simulink model "SO3_model_AIS"  (R2022a)
settings: Solver=ode4  StartTime=0.0  StopTime=180  FixedStep=0.02  RelTol=1e-3
values from neighbouring files (symbols this model uses):
  alpha = 0.05    [Ini_SO3.m]    (also in Ini_SO3_MixedCZ.m = 0.3; coneNew.m = acos(cosalpha))
  alpha1 = 0.25    [Ini_SO3.m]
  beta = 0.05    [Ini_SO3.m]    (also in Ini_SO3_MixedCZ.m = 0.3)
  deltar = 0.005    [Ini_SO3.m]    (also in Ini_SO3_MixedCZ.m = 0.01; Ini_Usat.m = 0.01)
  G = [1,0,0 ... (first row only)    [Ini_SO3.m]    (also in Ini_SO3_MixedCZ.m; Symmetric test.m = inv(J)*D*E*D')
  J0 = [60 0 -5 ... (first row only)    [Ini_SO3.m]    (also in Ini_SO3_MixedCZ.m)
  J1 = [60 0 -5 ... (first row only)    [Ini_SO3.m]    (also in Ini_SO3_MixedCZ.m)
  J2 = [60 0 -5 ... (first row only)    [Ini_SO3.m]    (also in Ini_SO3_MixedCZ.m)
  J3 = [60 0 -5 ... (first row only)    [Ini_SO3.m]    (also in Ini_SO3_MixedCZ.m)
  K1 = [0.01,0,30,0.2]'    [Ini_SO3.m]    (also in Ini_SO3_MixedCZ.m = [0.01,0,30,0.1]')
  K2 = [0.01,55,55,16,0.001,0.001,0.001]'    [Ini_SO3.m]
  lambda = 0.05    [Ini_SO3.m]    (also in Ini_SO3_MixedCZ.m = 0.3; SO3toThetan.m = diag(lambda))
  lambda1 = 0.25    [Ini_SO3.m]
  N = R/deltar    (= 200)    [Ini_SO3.m]    (also in Ini_SO3_MixedCZ.m; Ini_Usat.m)
  Omega01 = [0.03;0.02;-0.03]    [Ini_SO3.m]    (also in Ini_SO3_MixedCZ.m = [0,0,0])
  Omega02 = [-0.02;0.02;-0.03]    [Ini_SO3.m]    (also in Ini_SO3_MixedCZ.m = [0,0,0])
  Omega03 = [0;0.03;0.04]    [Ini_SO3.m]    (also in Ini_SO3_MixedCZ.m = [0,0,0])
  Omega0d = [0;0;0]    [Ini_SO3.m]    (also in Ini_SO3_MixedCZ.m)
  R = 1    [Ini_SO3.m]    (also in Ini_SO3_MixedCZ.m = 2; Ini_Usat.m = 2; SO3.m = eye(3)+(1-cos(ang))*x2x_hat(x)*x2x_hat(x)+sin(ang)*x2x_hat(x; plot2D.m = tran(lamda_con(j),phi_con(j)))
  R01 = SO3(deg2rad(-80), nd0)    [Ini_SO3.m]    (also in Ini_SO3_MixedCZ.m = SO3(2.387, [0.3145,0.9113,0.2658]'))
  R02 = SO3(deg2rad(40),[0;1;1]/norm([0;1;1]))    [Ini_SO3.m]    (also in Ini_SO3_MixedCZ.m = SO3(1.422, [0.1772,0.9751,-0.1329]'))
  R03 = SO3(deg2rad(-120), nd0)    [Ini_SO3.m]    (also in Ini_SO3_MixedCZ.m = SO3(2.007, [0.2997,0.9415,0.1543]'))
  Rd = SO3(-(2*pi-Angd),nd)    [Ini_SO3.m]    (also in Ini_SO3_MixedCZ.m = SO3(Angd,nd))
  Rd0 = SO3(-(2*pi-Angd0),nd0)    [Ini_SO3.m]    (also in Ini_SO3_MixedCZ.m = SO3(Angd0,nd0))
  thate_T = deg2rad(30)    [Ini_SO3.m]    (also in Ini_SO3_MixedCZ.m = deg2rad(10))
  X = zeros(4,4)    [Ini_SO3.m]    (also in Ini_SO3_MixedCZ.m; coneNew.m = R .* cos(A))
undefined symbols (not defined in the file or in its folder): deg, rad, s
libraries: matrix_library x7, aerolibconvert2 x5
(part 2 of 2)

== matlab function SO3_model_AIS/Virtual leader/Controller1 ==
  settings: updateMethod=DISCRETE
  data: Rd input; Omegad input; Omega1 input; R1 input; R10 input; G input; ud output; X input; alpha input; lambda input; K input; J1 input; Psit1 output; theta output; t input; dot_Phi1 output; a data_store_memory; b data_store_memory; tel_Id output; ant_Id output
function [ud,Psit1,theta,dot_Phi1,tel_Id,ant_Id]  = fcn(Rd,Omegad,Omega1,R1,R10,G,X,alpha,lambda,K,J1,t)
% X = n*4, 4= 1*3+1;
ud=zeros(3,1);
global a;
global b;

    %% Attitude Error Function
    
    Psit1 =0.5*trace(G*(eye(3)-Rd'*R1));
    
    e_R1t = x_hat2x(G*Rd'*R1-R1'*Rd*G);
    
    e_omega_1=Omega1-R1'*Rd*Omegad;
    
%     if t>70
%        aa=R1;
%     end
%     
    %% Attitude Error Dynamics

%     dot_Psit1 = e_omega_1'*e_R1t;
    dot_Psit1 = e_R1t;
    
    %% Mixed attitude constraints
%     tel = [0.750,0.433,0.500]'; %telescope
    tel = [0,0,1]'; %telescope
    ant = [0,1,0]'; %antenna
%     aa= R1*ant;
    tel_Id = zeros(3,1);
    ant_Id = zeros(3,1);
    
    tel_Id = R1*tel;
    ant_Id = R1*ant;
    
    
    Phi1 = 1;
    dot_Phi1 = zeros(3,1);
    n=(size(X,1));
    theta=zeros(4,1);
%         Ang=deg2rad(10);
        flag=zeros(4,1);

        for i = 1:n
            if i<n % static attitude-forbidden zones
                theta(i)=rad2deg(acos(tel'*R1'*X(i,1:3)'));
                    if b(i)==0
                        if cos(X(i,end))-tel'*R10'*X(i,1:3)'>0
                            a(i)=0;
                        end
                        if cos(X(i,end))-tel'*R10'*X(i,1:3)'<=0
                            a(i)=1;
                            if cos(X(i,end))-tel'*R1'*X(i,1:3)'>0 && abs(alpha*(tel'*R1'*X(i,1:3)'-cos(pi))^2/2+alpha * log((cos(X(i,end))-tel'*R1'*X(i,1:3)')/(1+cos(X(i,end)))))<0.01
                            a(i)=0;
                            b(i)=1;
                            end
                        end
                    end
                    if a(i)==1
                        Phi1=Phi1+alpha*(tel'*R1'*X(i,1:3)'-cos(pi))^2/2;
                        dot_Phi1 = dot_Phi1+alpha*(tel'*R1'*X(i,1:3)'-cos(pi))*(x2x_hat(R1'*X(i,1:3)')*tel);
                    else
                        Phi1 = Phi1  + (-alpha * log((cos(X(i,end))-tel'*R1'*X(i,1:3)')/(1+cos(X(i,end)))));
                        dot_Phi1 = dot_Phi1 ...
                        + (alpha*(x2x_hat(R1'*X(i,1:3)')*tel)/(tel'*R1'*X(i,1:3)'-cos(X(i,end))));
                    end    
             end
   
             if i==n % the attitude-mandatory zones
                 theta(i)=rad2deg(acos(ant'*R1'*X(i,1:3)'));
                    if b(i)==0
                        if cos(X(i,end))-ant'*R10'*X(i,1:3)'<0
                            a(i)=0;
                        end
                        if cos(X(i,end))-ant'*R10'*X(i,1:3)'>=0
                            a(i)=1;
                            if cos(X(i,end))-ant'*R1'*X(i,1:3)'<0 && abs(lambda*(cos(0)-ant'*R1'*X(i,1:3)')^2/2-(-lambda * log((ant'*R1'*X(i,1:3)'-cos(X(i,end)))/(1+cos(X(i,end))))))<0.01
                            a(i)=0;
                            b(i)=1;
                            end
                        end
                    end
                    if a(i)==1
                        Phi1 = Phi1 + lambda*(cos(0)-ant'*R1'*X(i,1:3)')^2/2;
                        dot_Phi1 = dot_Phi1-lambda *(cos(0)-ant'*R1'*X(i,1:3)')*(x2x_hat(R1'*X(i,1:3)')*ant);
                    else
                        Phi1 = Phi1  + (-lambda * log((ant'*R1'*X(i,1:3)'-cos(X(i,end)))/(1+cos(X(i,end)))));
                        dot_Phi1 = dot_Phi1 ...
                            + (lambda*(x2x_hat(R1'*X(i,1:3)')*ant)/(ant'*R1'*X(i,1:3)'-cos(X(i,end))));
                    end
            end
        end

% if flag==0 
%% 传统不考虑饱和控制器 
%         for i = 1:n
%                 if i<n % static attitude-forbidden zones
%                          Phi1 = Phi1  + (-alpha * log((cos(X(i,end))-tel'*R1'*X(i,1:3)')/(1+cos(X(i,end)))));
%                         dot_Phi1 = dot_Phi1 ...
%                         + (alpha*(x2x_hat(R1'*X(i,1:3)')*tel)/(tel'*R1'*X(i,1:3)'-cos(X(i,end))));
%                     theta(i)=rad2deg(acos(tel'*R1'*X(i,1:3)'));
%                 end
%                  if i==n % the attitude-mandatory zones
%                     theta(i)=rad2deg(acos(ant'*R1'*X(i,1:3)'));
%                         Phi1 = Phi1  + (-lambda * log((ant'*R1'*X(i,1:3)'-cos(X(i,end)))/(1+cos(X(i,end)))));
%                         dot_Phi1 = dot_Phi1 ...
%                             + (lambda*(x2x_hat(R1'*X(i,1:3)')*ant)/(ant'*R1'*X(i,1:3)'-cos(X(i,end))));
%                  end
%         end
%      if t>=300
        ksi=0.001; % 滑模平滑项
        S1=Omega1/((norm(Omega1)^2)+ksi);
        ud=-K(1)*Psit1*S1-K(3)*Omega1-K(4)*(Psit1*dot_Phi1+e_R1t*Phi1);
%      else
%         ud=[0,0,0]';
%      end
end

== matlab function SO3_model_AIS/Input saturation3/Sliding Mode Control2 ==
  data: s input; dot_hat_beta output; u input; hat_beta input
function dot_hat_beta  = fcn(s,u,hat_beta)
    dot_hat_beta=zeros(3,1);
   
   k_beta=0.05;
   ksi3 =1.1;
   delta3=0.001;
   
   if hat_beta(1)^2<ksi3 || (hat_beta(1)^2>=ksi3 && -s(1)*u(1)*hat_beta(1)<0)
        dot_hat_beta(1) = -k_beta*s(1)*u(1);
   end
   if hat_beta(1)^2>=ksi3 && -s(1)*u(1)*hat_beta(1)>=0
        dot_hat_beta(1) = k_beta*(-s(1)*u(1)-(norm(hat_beta(1))^2-ksi3)*(-s(1)*u(1))*hat_beta(1)/(delta3*norm(hat_beta(1))^2)*hat_beta(1));
   end
   
   if hat_beta(2)^2<ksi3 || (hat_beta(2)^2>=ksi3 && -s(2)*u(2)*hat_beta(2)<0)
        dot_hat_beta(2) = -k_beta*s(2)*u(2);
   end
   if hat_beta(2)^2>=ksi3 && -s(2)*u(2)*hat_beta(2)>=0
        dot_hat_beta(2) = k_beta*(-s(2)*u(2)-(norm(hat_beta(2))^2-ksi3)*(-s(2)*u(2))*hat_beta(2)/(delta3*norm(hat_beta(2))^2)*hat_beta(2));
   end
   
   if hat_beta(3)^2<ksi3 || (hat_beta(3)^2>=ksi3 && -s(3)*u(3)*hat_beta(3)<0)
        dot_hat_beta(3) = -k_beta*s(3)*u(3);
   end
   if hat_beta(3)^2>=ksi3 && -s(3)*u(3)*hat_beta(3)>=0
        dot_hat_beta(3) = k_beta*(-s(3)*u(3)-(norm(hat_beta(3))^2-ksi3)*(-s(3)*u(3))*hat_beta(3)/(delta3*norm(hat_beta(3))^2)*hat_beta(3));
   end


% 
% dot_hat_beta(1) = -k_beta*s(1)*u1(1);
% dot_hat_beta(2) = -k_beta*s(2)*u1(2);
% dot_hat_beta(3) = -k_beta*s(3)*u1(3);

== matlab function SO3_model_AIS/Input saturation3/Sliding Mode Control3 ==
  data: u_sat output; deltar input; hat_rou1 input; hat_rou2 input; hat_rou3 input; u input; t input; s input; dot_hat_rou1 output; dot_hat_rou2 output; dot_hat_rou3 output
function [u_sat,dot_hat_rou1,dot_hat_rou2,dot_hat_rou3]  = fcn(deltar,hat_rou1,hat_rou2,hat_rou3,u,t,s)
     N=200;
%      N=R/deltar;
%      N=max(N,R/deltar);
%      hat_rou=zeros(3,N);
     u_sat_temp=zeros(3,N);
     u_sat=zeros(3,1);
     
     k_rou=0.005;
    dot_hat_rou1 =zeros(N,1);
    dot_hat_rou2 =zeros(N,1);
    dot_hat_rou3 =zeros(N,1);
     if t==0
        dot_hat_rou1 =zeros(N,1);
        dot_hat_rou2 =zeros(N,1);
        dot_hat_rou3 =zeros(N,1);
     else
        for i=1:N
        dot_hat_rou1(i)=-k_rou*s(1)*DeadZone(i*deltar,u(1));
        dot_hat_rou2(i)=-k_rou*s(2)*DeadZone(i*deltar,u(2));
        dot_hat_rou3(i)=-k_rou*s(3)*DeadZone(i*deltar,u(3));
        end
     end
     
     if t==0
%         hat_rou=zeros(3,N); 
        u_sat=zeros(3,1);
     else
        for i=1:N
%          hat_rou(1,i)=deltat*dot_hat_rou(1,i)+hat_rou_old(1,i);
%          hat_rou(2,i)=deltat*dot_hat_rou(2,i)+hat_rou_old(2,i);
%          hat_rou(3,i)=deltat*dot_hat_rou(3,i)+hat_rou_old(3,i);
         u_sat_temp(1,i)= hat_rou1(i)*DeadZone(i*deltar,u(1));
         u_sat_temp(2,i)= hat_rou2(i)*DeadZone(i*deltar,u(2));
         u_sat_temp(3,i)= hat_rou3(i)*DeadZone(i*deltar,u(3));
%          u_sat_temp(1,i)= hat_rou(1,i);
%          u_sat_temp(2,i)= hat_rou(2,i);
%          u_sat_temp(3,i)= hat_rou(3,i);
        end
        u_sat(1)=sum(u_sat_temp(1,:))*deltar;
        u_sat(2)=sum(u_sat_temp(2,:))*deltar;
        u_sat(3)=sum(u_sat_temp(3,:))*deltar; 
     end
     
     
end

== matlab function SO3_model_AIS/Input saturation3/Sliding Mode Control5 ==
  data: u0 input; u1 output; hat_beta input; u_sat input
function u1  = fcn(u0,hat_beta,u_sat)
 u1=zeros(3,1);
 u1_temp=u0+u_sat;
u1(1)=hat_beta(1)*u1_temp(1);
u1(2)=hat_beta(2)*u1_temp(2);
u1(3)=hat_beta(3)*u1_temp(3);

== matlab function SO3_model_AIS/Input saturation3/Sliding Mode Control6 ==
  data: u1 input; w output; R input
function w  = fcn(u1,R)
    w=zeros(3,1);
    R=2*R;
    if u1(1)>=R
        w(1)=R/2;
    end
    if u1(1)>0 && u1(1)<R
        w(1)=u1(1)-1/R*1/2*u1(1)^2;
    end
    if u1(1)<=-R
        w(1)=-R/2;
    end
    if u1(1)<0 && u1(1)>-R
        w(1)=u1(1)+1/R*1/2*u1(1)^2;
    end
    %% 
    if u1(2)>=R
        w(2)=R/2;
    end
    if u1(2)>0 && u1(2)<R
        w(2)=u1(2)-1/R*1/2*u1(2)^2;
    end
    if u1(2)<=-R
        w(2)=-R/2;
    end
    if u1(2)<0 && u1(2)>-R
        w(2)=u1(2)+1/R*1/2*u1(2)^2;
    end
    
    %% 
    if u1(3)>=R
        w(3)=R/2;
    end
    if u1(3)>0 && u1(3)<R
        w(3)=u1(3)-1/R*1/2*u1(3)^2;
    end
    if u1(3)<=-R
        w(3)=-R/2;
    end
    if u1(3)<0 && u1(3)>-R
        w(3)=u1(3)+1/R*1/2*u1(3)^2;
    end
end

== matlab function SO3_model_AIS/Input saturation1/Sliding Mode Control2 ==
  data: s input; dot_hat_beta output; u input; hat_beta input
function dot_hat_beta  = fcn(s,u,hat_beta)
    dot_hat_beta=zeros(3,1);
   
   k_beta=0.05;
   ksi3 =1.1;
   delta3=0.001;
   
   if hat_beta(1)^2<ksi3 || (hat_beta(1)^2>=ksi3 && -s(1)*u(1)*hat_beta(1)<0)
        dot_hat_beta(1) = -k_beta*s(1)*u(1);
   end
   if hat_beta(1)^2>=ksi3 && -s(1)*u(1)*hat_beta(1)>=0
        dot_hat_beta(1) = k_beta*(-s(1)*u(1)-(norm(hat_beta(1))^2-ksi3)*(-s(1)*u(1))*hat_beta(1)/(delta3*norm(hat_beta(1))^2)*hat_beta(1));
   end
   
   if hat_beta(2)^2<ksi3 || (hat_beta(2)^2>=ksi3 && -s(2)*u(2)*hat_beta(2)<0)
        dot_hat_beta(2) = -k_beta*s(2)*u(2);
   end
   if hat_beta(2)^2>=ksi3 && -s(2)*u(2)*hat_beta(2)>=0
        dot_hat_beta(2) = k_beta*(-s(2)*u(2)-(norm(hat_beta(2))^2-ksi3)*(-s(2)*u(2))*hat_beta(2)/(delta3*norm(hat_beta(2))^2)*hat_beta(2));
   end
   
   if hat_beta(3)^2<ksi3 || (hat_beta(3)^2>=ksi3 && -s(3)*u(3)*hat_beta(3)<0)
        dot_hat_beta(3) = -k_beta*s(3)*u(3);
   end
   if hat_beta(3)^2>=ksi3 && -s(3)*u(3)*hat_beta(3)>=0
        dot_hat_beta(3) = k_beta*(-s(3)*u(3)-(norm(hat_beta(3))^2-ksi3)*(-s(3)*u(3))*hat_beta(3)/(delta3*norm(hat_beta(3))^2)*hat_beta(3));
   end


% 
% dot_hat_beta(1) = -k_beta*s(1)*u1(1);
% dot_hat_beta(2) = -k_beta*s(2)*u1(2);
% dot_hat_beta(3) = -k_beta*s(3)*u1(3);

== matlab function SO3_model_AIS/Input saturation1/Sliding Mode Control3 ==
  data: u_sat output; deltar input; hat_rou1 input; hat_rou2 input; hat_rou3 input; u input; t input; s input; dot_hat_rou1 output; dot_hat_rou2 output; dot_hat_rou3 output
function [u_sat,dot_hat_rou1,dot_hat_rou2,dot_hat_rou3]  = fcn(deltar,hat_rou1,hat_rou2,hat_rou3,u,t,s)
     N=200;
%      N=R/deltar;
%      N=max(N,R/deltar);
%      hat_rou=zeros(3,N);
     u_sat_temp=zeros(3,N);
     u_sat=zeros(3,1);
     
     k_rou=0.005;
    dot_hat_rou1 =zeros(N,1);
    dot_hat_rou2 =zeros(N,1);
    dot_hat_rou3 =zeros(N,1);
     if t==0
        dot_hat_rou1 =zeros(N,1);
        dot_hat_rou2 =zeros(N,1);
        dot_hat_rou3 =zeros(N,1);
     else
        for i=1:N
        dot_hat_rou1(i)=k_rou*s(1)*DeadZone(i*deltar,u(1));
        dot_hat_rou2(i)=k_rou*s(2)*DeadZone(i*deltar,u(2));
        dot_hat_rou3(i)=k_rou*s(3)*DeadZone(i*deltar,u(3));
        end
     end
     
     if t==0
%         hat_rou=zeros(3,N); 
        u_sat=zeros(3,1);
     else
        for i=1:N
%          hat_rou(1,i)=deltat*dot_hat_rou(1,i)+hat_rou_old(1,i);
%          hat_rou(2,i)=deltat*dot_hat_rou(2,i)+hat_rou_old(2,i);
%          hat_rou(3,i)=deltat*dot_hat_rou(3,i)+hat_rou_old(3,i);
         u_sat_temp(1,i)= hat_rou1(i)*DeadZone(i*deltar,u(1));
         u_sat_temp(2,i)= hat_rou2(i)*DeadZone(i*deltar,u(2));
         u_sat_temp(3,i)= hat_rou3(i)*DeadZone(i*deltar,u(3));
%          u_sat_temp(1,i)= hat_rou(1,i);
%          u_sat_temp(2,i)= hat_rou(2,i);
%          u_sat_temp(3,i)= hat_rou(3,i);
        end
        u_sat(1)=sum(u_sat_temp(1,:))*deltar;
        u_sat(2)=sum(u_sat_temp(2,:))*deltar;
        u_sat(3)=sum(u_sat_temp(3,:))*deltar; 
     end
     
     
end

== matlab function SO3_model_AIS/Input saturation1/Sliding Mode Control5 ==
  data: u0 input; u1 output; hat_beta input; u_sat input
function u1  = fcn(u0,hat_beta,u_sat)
 u1=zeros(3,1);
 u1_temp=u0-u_sat;
u1(1)=hat_beta(1)*u1_temp(1);
u1(2)=hat_beta(2)*u1_temp(2);
u1(3)=hat_beta(3)*u1_temp(3);

== matlab function SO3_model_AIS/Input saturation1/Sliding Mode Control6 ==
  data: u1 input; w output; R input
function w  = fcn(u1,R)
    w=zeros(3,1);
     R=2*R;
    if u1(1)>=R
        w(1)=R/2;
    end
    if u1(1)>0 && u1(1)<R
        w(1)=u1(1)-1/R*1/2*u1(1)^2;
    end
    if u1(1)<=-R
        w(1)=-R/2;
    end
    if u1(1)<0 && u1(1)>-R
        w(1)=u1(1)+1/R*1/2*u1(1)^2;
    end
    %% 
    if u1(2)>=R
        w(2)=R/2;
    end
    if u1(2)>0 && u1(2)<R
        w(2)=u1(2)-1/R*1/2*u1(2)^2;
    end
    if u1(2)<=-R
        w(2)=-R/2;
    end
    if u1(2)<0 && u1(2)>-R
        w(2)=u1(2)+1/R*1/2*u1(2)^2;
    end
    
    %% 
    if u1(3)>=R
        w(3)=R/2;
    end
    if u1(3)>0 && u1(3)<R
        w(3)=u1(3)-1/R*1/2*u1(3)^2;
    end
    if u1(3)<=-R
        w(3)=-R/2;
    end
    if u1(3)<0 && u1(3)>-R
        w(3)=u1(3)+1/R*1/2*u1(3)^2;
    end
end

== matlab function SO3_model_AIS/Input saturation2/Sliding Mode Control2 ==
  data: s input; dot_hat_beta output; u input; hat_beta input
function dot_hat_beta  = fcn(s,u,hat_beta)
    dot_hat_beta=zeros(3,1);
   
   k_beta=0.05;
   ksi3 =1.1;
   delta3=0.001;
   
   if hat_beta(1)^2<ksi3 || (hat_beta(1)^2>=ksi3 && -s(1)*u(1)*hat_beta(1)<0)
        dot_hat_beta(1) = -k_beta*s(1)*u(1);
   end
   if hat_beta(1)^2>=ksi3 && -s(1)*u(1)*hat_beta(1)>=0
        dot_hat_beta(1) = k_beta*(-s(1)*u(1)-(norm(hat_beta(1))^2-ksi3)*(-s(1)*u(1))*hat_beta(1)/(delta3*norm(hat_beta(1))^2)*hat_beta(1));
   end
   
   if hat_beta(2)^2<ksi3 || (hat_beta(2)^2>=ksi3 && -s(2)*u(2)*hat_beta(2)<0)
        dot_hat_beta(2) = -k_beta*s(2)*u(2);
   end
   if hat_beta(2)^2>=ksi3 && -s(2)*u(2)*hat_beta(2)>=0
        dot_hat_beta(2) = k_beta*(-s(2)*u(2)-(norm(hat_beta(2))^2-ksi3)*(-s(2)*u(2))*hat_beta(2)/(delta3*norm(hat_beta(2))^2)*hat_beta(2));
   end
   
   if hat_beta(3)^2<ksi3 || (hat_beta(3)^2>=ksi3 && -s(3)*u(3)*hat_beta(3)<0)
        dot_hat_beta(3) = -k_beta*s(3)*u(3);
   end
   if hat_beta(3)^2>=ksi3 && -s(3)*u(3)*hat_beta(3)>=0
        dot_hat_beta(3) = k_beta*(-s(3)*u(3)-(norm(hat_beta(3))^2-ksi3)*(-s(3)*u(3))*hat_beta(3)/(delta3*norm(hat_beta(3))^2)*hat_beta(3));
   end

% dot_hat_beta(1) = -k_beta*s(1)*u1(1);
% dot_hat_beta(2) = -k_beta*s(2)*u1(2);
% dot_hat_beta(3) = -k_beta*s(3)*u1(3);

== matlab function SO3_model_AIS/Input saturation2/Sliding Mode Control3 ==
  data: u_sat output; deltar input; hat_rou1 input; hat_rou2 input; hat_rou3 input; u input; t input; s input; dot_hat_rou1 output; dot_hat_rou2 output; dot_hat_rou3 output
function [u_sat,dot_hat_rou1,dot_hat_rou2,dot_hat_rou3]  = fcn(deltar,hat_rou1,hat_rou2,hat_rou3,u,t,s)
     N=200;
%      N=R/deltar;
%      N=max(N,R/deltar);
%      hat_rou=zeros(3,N);
     u_sat_temp=zeros(3,N);
     u_sat=zeros(3,1);
     
     k_rou=0.005;
    dot_hat_rou1 =zeros(N,1);
    dot_hat_rou2 =zeros(N,1);
    dot_hat_rou3 =zeros(N,1);
     if t==0
        dot_hat_rou1 =zeros(N,1);
        dot_hat_rou2 =zeros(N,1);
        dot_hat_rou3 =zeros(N,1);
     else
        for i=1:N
        dot_hat_rou1(i)=k_rou*s(1)*DeadZone(i*deltar,u(1));
        dot_hat_rou2(i)=k_rou*s(2)*DeadZone(i*deltar,u(2));
        dot_hat_rou3(i)=k_rou*s(3)*DeadZone(i*deltar,u(3));
        end
     end
     
     if t==0
%         hat_rou=zeros(3,N); 
        u_sat=zeros(3,1);
     else
        for i=1:N
%          hat_rou(1,i)=deltat*dot_hat_rou(1,i)+hat_rou_old(1,i);
%          hat_rou(2,i)=deltat*dot_hat_rou(2,i)+hat_rou_old(2,i);
%          hat_rou(3,i)=deltat*dot_hat_rou(3,i)+hat_rou_old(3,i);
         u_sat_temp(1,i)= hat_rou1(i)*DeadZone(i*deltar,u(1));
         u_sat_temp(2,i)= hat_rou2(i)*DeadZone(i*deltar,u(2));
         u_sat_temp(3,i)= hat_rou3(i)*DeadZone(i*deltar,u(3));
%          u_sat_temp(1,i)= hat_rou(1,i);
%          u_sat_temp(2,i)= hat_rou(2,i);
%          u_sat_temp(3,i)= hat_rou(3,i);
        end
        u_sat(1)=sum(u_sat_temp(1,:))*deltar;
        u_sat(2)=sum(u_sat_temp(2,:))*deltar;
        u_sat(3)=sum(u_sat_temp(3,:))*deltar; 
     end
     
     
end

== matlab function SO3_model_AIS/Input saturation2/Sliding Mode Control5 ==
  data: u0 input; u1 output; hat_beta input; u_sat input
function u1  = fcn(u0,hat_beta,u_sat)
 u1=zeros(3,1);
 u1_temp=u0-u_sat;
u1(1)=hat_beta(1)*u1_temp(1);
u1(2)=hat_beta(2)*u1_temp(2);
u1(3)=hat_beta(3)*u1_temp(3);

== matlab function SO3_model_AIS/Input saturation2/Sliding Mode Control6 ==
  data: u1 input; w output; R input
function w  = fcn(u1,R)
    w=zeros(3,1);
    R=2*R;
    if u1(1)>=R
        w(1)=R/2;
    end
    if u1(1)>0 && u1(1)<R
        w(1)=u1(1)-1/R*1/2*u1(1)^2;
    end
    if u1(1)<=-R
        w(1)=-R/2;
    end
    if u1(1)<0 && u1(1)>-R
        w(1)=u1(1)+1/R*1/2*u1(1)^2;
    end
    %% 
    if u1(2)>=R
        w(2)=R/2;
    end
    if u1(2)>0 && u1(2)<R
        w(2)=u1(2)-1/R*1/2*u1(2)^2;
    end
    if u1(2)<=-R
        w(2)=-R/2;
    end
    if u1(2)<0 && u1(2)>-R
        w(2)=u1(2)+1/R*1/2*u1(2)^2;
    end
    
    %% 
    if u1(3)>=R
        w(3)=R/2;
    end
    if u1(3)>0 && u1(3)<R
        w(3)=u1(3)-1/R*1/2*u1(3)^2;
    end
    if u1(3)<=-R
        w(3)=-R/2;
    end
    if u1(3)<0 && u1(3)>-R
        w(3)=u1(3)+1/R*1/2*u1(3)^2;
    end
end

== matlab function SO3_model_AIS/Virtual leader/MATLAB Function1 ==
  data: R input; n output; theta output; aa output
function [n,theta,aa]   = fcn(R)
    %So3 到轴角
    n=zeros(3,1);
    theta=0;
    
    n=zeros(3,1);
    theta=0;
    aa=0;
    theta=acos((trace(R)-1)/2);
    [A,lambda]=eig(R);
    lambda=real(lambda);
    lambda=diag(lambda);
    a=1;
    for i=1:3
        if lambda(i)>=0.99
            a=i;
            aa=1;
        end
    end
    b=a;
    n_temp=A(:,b);
    n_temp=n_temp/norm(n_temp);
    n1=real(n_temp(1));
    n2=real(n_temp(2));
    n3=real(n_temp(3));
   n=[n1;n2;n3];
end

== matlab function SO3_model_AIS/Controller/Controller1 ==
  settings: updateMethod=DISCRETE
  data: R1 input; R2 input; R3 input; Omega1 input; Omega2 input; Omega3 input; Rd input; Omegad input; R10 input; R20 input; R30 input; G input; u10_nod output; u20_nod output; u30_nod output; Psi output; t input; Psit output; Psic output; X input; thate_T input; norm_e_omega output; alpha input; lambda input; beta input; K input; theta_1 output; theta_12 output; theta_13 output; theta_2 output; theta_21 output; theta_23 output; theta_3 output; theta_31 output; theta_32 output; tel_I1 output; ant_I1 output; tel_I2 output; ant_I2 output; tel_I3 output; ant_I3 output; SFZ2 output; SMZ1 output
function [u10_nod,u20_nod,u30_nod,Psi,Psit,Psic,norm_e_omega,theta_1,theta_12,...
    theta_13,theta_2,theta_21,theta_23,theta_3,theta_31,theta_32,...
    tel_I1,ant_I1,tel_I2,ant_I2,tel_I3,ant_I3,SFZ2,SMZ1]...
    = fcn(R1,R2,R3,Omega1,Omega2,Omega3,Rd,Omegad,R10,R20,R30,G,t,X,thate_T,alpha,lambda,beta,K)
% X = n*4, 4= 1*3+1;
    %% Attitude Error Function
    u10_nod=zeros(3,1);
    u20_nod=zeros(3,1);
    u30_nod=zeros(3,1);
    Psi=zeros(3,1);
    Psit=zeros(3,1);
    Psic=zeros(3,1);
    norm_e_omega=zeros(3,1);
    
    Psit1 =0.5*trace(G*(eye(3)-Rd'*R1));
    Psit2 =0.5*trace(G*(eye(3)-Rd'*R2));
    Psit3 =0.5*trace(G*(eye(3)-Rd'*R3));
    Psit = [Psit1;Psit2;Psit3];
    
    Psic1 =0.5*trace(G*(eye(3)-R3'*R1))+0.5*trace(G*(eye(3)-R2'*R1));
    Psic2 =0.5*trace(G*(eye(3)-R1'*R2))+0.5*trace(G*(eye(3)-R3'*R2));
    Psic3 =0.5*trace(G*(eye(3)-R2'*R3))+0.5*trace(G*(eye(3)-R1'*R3));
    Psic = [Psic1;Psic2;Psic3];
    
    Psi1 = Psit1+Psic1;
    Psi2 = Psic2;
    Psi3 = Psic3;
    
    Psi = [Psi1;Psi2;Psi3];
    
    e_R12c=x_hat2x(G*R2'*R1-R1'*R2*G);
    e_R13c=x_hat2x(G*R3'*R1-R1'*R3*G);
    e_R1c = e_R12c+e_R13c;
    e_R1t = x_hat2x(G*Rd'*R1-R1'*Rd*G);
    e_R1 = e_R1c+e_R1t;
    
    e_R21c=x_hat2x(G*R1'*R2-R2'*R1*G);
    e_R23c=x_hat2x(G*R3'*R2-R2'*R3*G);
    e_R2c = e_R21c+e_R23c;
    e_R2t = 0*x_hat2x(G*Rd'*R2-R2'*Rd*G);
    e_R2 = e_R2c+e_R2t;
    
    e_R31c=x_hat2x(G*R1'*R3-R3'*R1*G);
    e_R32c=x_hat2x(G*R2'*R3-R3'*R2*G);
    e_R3c = e_R31c+e_R32c;
    e_R3t = 0*x_hat2x(G*Rd'*R3-R3'*Rd*G);
    e_R3 = e_R3c+e_R3t;
    
    e_omega_c_12=Omega1-R1'*R2*Omega2;
    e_omega_c_13=Omega1-R1'*R3*Omega3;
    e_omega_c_1=e_omega_c_12+e_omega_c_13;
    e_omega_t_1=Omega1-R1'*Rd*Omegad;
    e_omega_1 = e_omega_c_1+e_omega_t_1;
    
    e_omega_c_21=Omega2-R2'*R1*Omega1;
    e_omega_c_23=Omega2-R2'*R3*Omega3;
    e_omega_c_2=e_omega_c_21+e_omega_c_23;
    e_omega_t_2=Omega2-R2'*Rd*Omegad;
    e_omega_2 = e_omega_c_2+e_omega_t_2;
    
    e_omega_c_31=Omega3-R3'*R1*Omega1;
    e_omega_c_32=Omega3-R3'*R2*Omega2;
    e_omega_c_3=e_omega_c_31+e_omega_c_32;
    e_omega_t_3=Omega3-R3'*Rd*Omegad;
    e_omega_3 = e_omega_c_3+e_omega_t_3;
    
    norm_e_omega=[norm(e_omega_1);norm(e_omega_2);norm(e_omega_3)];
    
    %% Attitude Error Dynamics
%     dot_Psic1 = e_omega_c_12'*e_R12c+e_omega_c_13'*e_R13c;
%     dot_Psit1 = e_omega_t_1'*e_R1t;
%     dot_Psi1 = dot_Psic1+dot_Psit1;
%     
%     dot_Psic2 = e_omega_c_21'*e_R21c+e_omega_c_23'*e_R23c;
%     dot_Psit2 = e_omega_t_2'*e_R2t;
%     dot_Psi2 = dot_Psic2+dot_Psit2;
%     
%     dot_Psic3 = e_omega_c_31'*e_R31c+e_omega_c_31'*e_R32c;
%     dot_Psit3 = e_omega_t_3'*e_R3t;
%     dot_Psi3 = dot_Psic3+dot_Psit3;
    
    %% Mixed attitude constraints
%     tel = [0.750,0.433,0.500]'; %telescope
%     tel = [0,0,1]'; %telescope
%     ant = [0,1,0]'; %antenna

% tel = [0.750,0.433,0.500]'; %telescope
    tel = [0,0,1]'; %telescope
    ant = [0,1,0]'; %antenna
%     tru= [-1,0,0;0,-1,0;0,0,-1]';  %three trust
tru= [-1,0,0;0,-1,0;0.750,0.433,0.500]';  %three trust
    
    tel_Id = zeros(3,1);
    ant_Id = zeros(3,1);
    
    tel_I1 = zeros(3,1);
    ant_I1 = zeros(3,1);
    
    tel_I2 = zeros(3,1);
    ant_I2 = zeros(3,1);
    
    tel_I3 = zeros(3,1);
    ant_I3 = zeros(3,1);
    
    tel_Id = Rd*tel;
    ant_Id = Rd*ant;
    
    tel_I1 = R1*tel;
    ant_I1 = R1*ant;
    
    tel_I2 = R2*tel;
    ant_I2 = R2*ant;
    
    tel_I3 = R3*tel;
    ant_I3 = R3*ant;
    
    
    Phi1 = 1;
    P_Phi1 = zeros(3,1);
    Phi2 = 1;
    P_Phi2 = zeros(3,1);
    Phi3 = 1;
    P_Phi3 = zeros(3,1);
    n=(size(X,1)+1);
    
    P_DF1=0;
    P_DF2=0;
    P_DF3=0;
    theta_1=zeros(4,1);
    theta_12=zeros(3,1);
    theta_13=zeros(3,1);
    
    theta_2=zeros(4,1);
    theta_21=zeros(3,1);
    theta_23=zeros(3,1);
    
    theta_3=zeros(4,1);
    theta_31=zeros(3,1);
    theta_32=zeros(3,1);
    
for i = 1:n
    if i<n-1 % static attitude-forbidden zones
         if (cos(X(i,end))-tel'*R10'*X(i,1:3)')>0
         Phi1 = Phi1  + (-alpha * log((cos(X(i,end))-tel'*R1'*X(i,1:3)')/(1+cos(X(i,end)))));
         P_Phi1 = P_Phi1 ...
                          + (alpha*(x2x_hat(R1'*X(i,1:3)')*tel)/(tel'*R1'*X(i,1:3)'-cos(X(i,end))));
         else
         Phi1=Phi1+alpha*(tel'*R1'*X(i,1:3)'-cos(pi))^2/2;
         P_Phi1 = P_Phi1+alpha*(tel'*R1'*X(i,1:3)'-cos(pi))*(x2x_hat(R1'*X(i,1:3)')*tel);
         end
        theta_1(i)=rad2deg(acos(tel'*R1'*X(i,1:3)'));
       
        if (cos(X(i,end))-tel'*R20'*X(i,1:3)')>0
            Phi2 = Phi2  + (-alpha * log((cos(X(i,end))-tel'*R2'*X(i,1:3)')/(1+cos(X(i,end)))));
            P_Phi2 = P_Phi2 ...
                + (alpha*(x2x_hat(R2'*X(i,1:3)')*tel)/(tel'*R2'*X(i,1:3)'-cos(X(i,end))));
        else
             Phi2=Phi2+alpha*(tel'*R2'*X(i,1:3)'-cos(pi))^2/2;
             P_Phi2 = P_Phi2+alpha*(tel'*R2'*X(i,1:3)'-cos(pi))*(x2x_hat(R2'*X(i,1:3)')*tel);
        end
        
        theta_2(i)=rad2deg(acos(tel'*R2'*X(i,1:3)'));
        
        
        if (cos(X(i,end))-tel'*R30'*X(i,1:3)')>0
            Phi3 = Phi3  + (-alpha * log((cos(X(i,end))-tel'*R3'*X(i,1:3)')/(1+cos(X(i,end)))));
            P_Phi3 = P_Phi3 ...
                + (alpha*(x2x_hat(R3'*X(i,1:3)')*tel)/(tel'*R3'*X(i,1:3)'-cos(X(i,end))));
        else
            Phi3=Phi3+alpha*(tel'*R3'*X(i,1:3)'-cos(pi))^2/2;
             P_Phi3 = P_Phi3-alpha*(tel'*R3'*X(i,1:3)'-cos(pi))*(x2x_hat(R3'*X(i,1:3)')*tel);
        end
         theta_3(i)=rad2deg(acos(tel'*R3'*X(i,1:3)'));
    end
    if i==n-1 % the attitude-mandatory zones
        
        if (ant'*R10'*X(i,1:3)'-cos(X(i,end)))>0
            Phi1 = Phi1  + (-lambda * log((ant'*R1'*X(i,1:3)'-cos(X(i,end)))/(1+cos(X(i,end)))));
            P_Phi1 = P_Phi1 ...
                + (lambda*(x2x_hat(R1'*X(i,1:3)')*ant)/(ant'*R1'*X(i,1:3)'-cos(X(i,end))));
        else
            Phi1 = Phi1 + lambda*(cos(0)-ant'*R1'*X(i,1:3)')^2/2;
            P_Phi1 = P_Phi1-lambda *(cos(0)-ant'*R1'*X(i,1:3)')*(x2x_hat(R1'*X(i,1:3)')*ant);
        end    
        theta_1(i)=rad2deg(acos(ant'*R1'*X(i,1:3)'));
        
        if (ant'*R20'*X(i,1:3)'-cos(X(i,end)))>0
            Phi2 = Phi2  + (-lambda * log((ant'*R2'*X(i,1:3)'-cos(X(i,end)))/(1+cos(X(i,end)))));
            P_Phi2 = P_Phi2 ...
                + (lambda*(x2x_hat(R2'*X(i,1:3)')*ant)/(ant'*R2'*X(i,1:3)'-cos(X(i,end))));
        else
            Phi2 = Phi2 + lambda*(cos(0)-ant'*R2'*X(i,1:3)')^2/2;
            P_Phi2 = P_Phi2-lambda *(cos(0)-ant'*R2'*X(i,1:3)')*(x2x_hat(R2'*X(i,1:3)')*ant);
        end
        theta_2(i)=rad2deg(acos(ant'*R2'*X(i,1:3)'));
        
        if (ant'*R30'*X(i,1:3)'-cos(X(i,end)))>0
        Phi3 = Phi3  + (-lambda * log((ant'*R3'*X(i,1:3)'-cos(X(i,end)))/(1+cos(X(i,end)))));
        P_Phi3 = P_Phi3 ...
            + (lambda*(x2x_hat(R3'*X(i,1:3)')*ant)/(ant'*R3'*X(i,1:3)'-cos(X(i,end))));
        else
        Phi3 = Phi3 + lambda*(cos(0)-ant'*R3'*X(i,1:3)')^2/2;
        P_Phi3 = P_Phi3-lambda *(cos(0)-ant'*R3'*X(i,1:3)')*(x2x_hat(R3'*X(i,1:3)')*ant);
        end
        theta_3(i)=rad2deg(acos(ant'*R3'*X(i,1:3)'));
    end
    if i==n % relative dynamic attitude-forbidden zones
        for j=1:3 % three trust
            
            if (cos(thate_T)-tel'*R10'*R20*tru(j,:)')>0
                Phi1 = Phi1  + (-beta * log((cos(thate_T)-tel'*R1'*R2*tru(j,:)')/(1+cos(thate_T))));
                P_Phi1 = P_Phi1 ...
                    + (beta*(x2x_hat(R1'*R2*tru(j,:)')*tel)/(tel'*R1'*R2*tru(j,:)'-cos(thate_T)));
                P_DF1= P_DF1+ (R1'*R2*Omega2)'*(beta*(x2x_hat(R1'*R2*tru(j,:)')*tel)/(tel'*R1'*R2*tru(j,:)'-cos(thate_T)));
            else
                Phi1 = Phi1  + beta *((tel'*R1'*R2*tru(j,:)'-cos(pi))^2/2);
                P_Phi1 = P_Phi1- (beta*(tel'*R1'*R2*tru(j,:)'-cos(pi))*(x2x_hat(R1'*R2*tru(j,:)')*tel));
                P_DF1= P_DF1+ (R1'*R2*Omega2)'*(-(beta*(tel'*R1'*R2*tru(j,:)'-cos(pi))*(x2x_hat(R1'*R2*tru(j,:)')*tel)));
            end
            
            if (cos(thate_T)-tel'*R10'*R30*tru(j,:)')>0
                Phi1 = Phi1  + (-beta * log((cos(thate_T)-tel'*R1'*R3*tru(j,:)')/(1+cos(thate_T))));
                P_Phi1 = P_Phi1 ...
                    + (beta*(x2x_hat(R1'*R3*tru(j,:)')*tel)/(tel'*R1'*R3*tru(j,:)'-cos(thate_T)));
                P_DF1= P_DF1+ (R1'*R3*Omega3)'*(beta*(x2x_hat(R1'*R3*tru(j,:)')*tel)/(tel'*R1'*R3*tru(j,:)'-cos(thate_T)));
            else
                Phi1 = Phi1  + beta *((tel'*R1'*R3*tru(j,:)'-cos(pi))^2/2);
                P_Phi1 = P_Phi1- (beta*(tel'*R1'*R3*tru(j,:)'-cos(pi))*(x2x_hat(R1'*R3*tru(j,:)')*tel));
                P_DF1= P_DF1+ (R1'*R3*Omega3)'*(-(beta*(tel'*R1'*R3*tru(j,:)'-cos(pi))*(x2x_hat(R1'*R3*tru(j,:)')*tel)));
            end
            
%             theta_12(j)=rad2deg(acos(tel'*R1'*R2*tru(j,:)'));
%             theta_13(j)=rad2deg(acos(tel'*R1'*R3*tru(j,:)'));       
            if abs(tel'*R1'*R2*tru(j,:)')>1
               theta_12(j)=rad2deg(acos(sign(tel'*R1'*R2*tru(j,:)'))); 
            else
               theta_12(j)=rad2deg(acos(tel'*R1'*R2*tru(j,:)'));
            end
            if abs(tel'*R1'*R3*tru(j,:)')>1
               theta_13(j)=rad2deg(acos(sign(tel'*R1'*R3*tru(j,:)'))); 
            else
               theta_13(j)=rad2deg(acos(tel'*R1'*R3*tru(j,:)'));
            end        
                   
%             if (cos(thate_T)-tel'*R20'*R10*tru(j,:)')>0
%                 Phi2 = Phi2  + (-beta * log((cos(thate_T)-tel'*R2'*R1*tru(j,:)')/(1+cos(thate_T))));
%                 P_Phi2 = P_Phi2 ...
%                     + (beta*(x2x_hat(R2'*R1*tru(j,:)')*tel)/(tel'*R2'*R1*tru(j,:)'-cos(thate_T)));
%                 P_DF2= P_DF2+ (R2'*R1*Omega1)'*(beta*(x2x_hat(R2'*R1*tru(j,:)')*tel)/(tel'*R2'*R1*tru(j,:)'-cos(thate_T)));
%             else
                Phi2 = Phi2  + beta *((tel'*R2'*R1*tru(j,:)'-cos(pi))^2/2);
                P_Phi2 = P_Phi2- (beta*(tel'*R2'*R1*tru(j,:)'-cos(pi))*(x2x_hat(R2'*R1*tru(j,:)')*tel));
                P_DF2= P_DF2+ (R2'*R1*Omega1)'*(-(beta*(tel'*R2'*R1*tru(j,:)'-cos(pi))*(x2x_hat(R2'*R1*tru(j,:)')*tel)));
%             end

            if (cos(thate_T)-tel'*R20'*R30*tru(j,:)')>0
                Phi2 = Phi2  + (-beta * log((cos(thate_T)-tel'*R2'*R3*tru(j,:)')/(1+cos(thate_T))));
                P_Phi2 = P_Phi2 ...
                    + (beta*(x2x_hat(R2'*R3*tru(j,:)')*tel)/(tel'*R2'*R3*tru(j,:)'-cos(thate_T)));
                P_DF2= P_DF2+ (R2'*R3*Omega3)'*(beta*(x2x_hat(R2'*R3*tru(j,:)')*tel)/(tel'*R2'*R3*tru(j,:)'-cos(thate_T)));
            else
                Phi2 = Phi2  + beta *((tel'*R2'*R3*tru(j,:)'-cos(pi))^2/2);
                P_Phi2 = P_Phi2- (beta*(tel'*R2'*R3*tru(j,:)'-cos(pi))*(x2x_hat(R2'*R3*tru(j,:)')*tel));
                P_DF2= P_DF2+ (R2'*R3*Omega3)'*(-(beta*(tel'*R2'*R3*tru(j,:)'-cos(pi))*(x2x_hat(R2'*R3*tru(j,:)')*tel)));
            end
             
%             theta_21(j)=rad2deg(acos(tel'*R2'*R1*tru(j,:)'));
%             theta_23(j)=rad2deg(acos(tel'*R2'*R3*tru(j,:)'));
            
            if abs(tel'*R2'*R1*tru(j,:)')>1
               theta_21(j)=rad2deg(acos(sign(tel'*R2'*R1*tru(j,:)'))); 
            else
                theta_21(j)=rad2deg(acos(tel'*R2'*R1*tru(j,:)'));
            end
            if abs(tel'*R3'*R2*tru(j,:)')>1
               theta_23(j)=rad2deg(acos(sign(tel'*R3'*R2*tru(j,:)'))); 
            else
               theta_23(j)=rad2deg(acos(tel'*R2'*R3*tru(j,:)'));
            end       
                   
%              if (cos(thate_T)-tel'*R30'*R10*tru(j,:)')>0
%                 Phi3 = Phi3  + (-beta * log((cos(thate_T)-tel'*R3'*R1*tru(j,:)')/(1+cos(thate_T))));
%                 P_Phi3 = P_Phi3 ...
%                     + (beta*(x2x_hat(R3'*R1*tru(j,:)')*tel)/(tel'*R3'*R1*tru(j,:)'-cos(thate_T)));
%                 P_DF3= P_DF3+ (R3'*R1*Omega1)'*(beta*(x2x_hat(R3'*R1*tru(j,:)')*tel)/(tel'*R3'*R1*tru(j,:)'-cos(thate_T)));
%             else
                Phi3 = Phi3  + beta *((tel'*R3'*R1*tru(j,:)'-cos(pi))^2/2);
                P_Phi3 = P_Phi3- (beta*(tel'*R3'*R1*tru(j,:)'-cos(pi))*(x2x_hat(R3'*R1*tru(j,:)')*tel));
                P_DF3= P_DF3+ (R3'*R1*Omega1)'*(-(beta*(tel'*R3'*R1*tru(j,:)'-cos(pi))*(x2x_hat(R3'*R1*tru(j,:)')*tel)));
%              end

            if (cos(thate_T)-tel'*R30'*R20*tru(j,:)')>0
                Phi3 = Phi3  + (-beta * log((cos(thate_T)-tel'*R3'*R2*tru(j,:)')/(1+cos(thate_T))));
                P_Phi3 = P_Phi3 ...
                    + (beta*(x2x_hat(R3'*R2*tru(j,:)')*tel)/(tel'*R3'*R2*tru(j,:)'-cos(thate_T)));
                P_DF3= P_DF3+ (R3'*R2*Omega2)'*(beta*(x2x_hat(R3'*R2*tru(j,:)')*tel)/(tel'*R3'*R2*tru(j,:)'-cos(thate_T)));
            else
                Phi3 = Phi3  + beta *((tel'*R3'*R2*tru(j,:)'-cos(pi))^2/2);
                P_Phi3 = P_Phi3- (beta*(tel'*R3'*R2*tru(j,:)'-cos(pi))*(x2x_hat(R3'*R2*tru(j,:)')*tel));
                P_DF3= P_DF3+ (R3'*R2*Omega2)'*(-(beta*(tel'*R3'*R2*tru(j,:)'-cos(pi))*(x2x_hat(R3'*R2*tru(j,:)')*tel)));
            end
            if abs(tel'*R3'*R1*tru(j,:)')>1
               theta_31(j)=rad2deg(acos(sign(tel'*R3'*R1*tru(j,:)'))); 
            else
                theta_31(j)=rad2deg(acos(tel'*R3'*R1*tru(j,:)'));
            end
            if abs(tel'*R3'*R2*tru(j,:)')>1
               theta_32(j)=rad2deg(acos(sign(tel'*R3'*R2*tru(j,:)'))); 
            else
                theta_32(j)=rad2deg(acos(tel'*R3'*R2*tru(j,:)'));
            end
        end
    end
end

SFZ2=[theta_1(2);theta_2(2);theta_3(2)];
SMZ1=[theta_1(4);theta_2(4);theta_3(4)];

%% 传统不考虑饱和控制器
ksi=0.01; % 滑模平滑项
% if t>400
%     K(4)=0.01;
% end
S1=Omega1/((norm(Omega1))^2+ksi);
S11=Omega1/((norm(Omega1))+ksi);
F1=e_R1*Phi1+Psi1*P_Phi1;
A1=(R1'*R2*Omega2)'*e_R12c+(R1'*R3*Omega3)'*e_R13c;
% u10=-K(1)*Psic1*S1-K(2)*Psit1*S1-K(3)*(e_omega_1)'*e_omega_1*S1+2*K(3)*e_omega_c_1'*e_omega_t_1*S1...
%     -K(4)*F1+K(4)*Psi1*P_DF1*S1+K(4)*Phi1*A1*S1+K(4)*Phi1*((R1'*Rd*Omegad)'*e_R1t)*S1; %no disturbence
u10_nod=-K(1)*Psi1*S1-K(2)*norm(e_omega_1)*S11-K(3)*(e_omega_1)...
    -K(4)*F1+K(4)*Psi1*P_DF1*S1+K(4)*Phi1*A1*S1+K(4)*Phi1*((R1'*Rd*Omegad)'*e_R1t)*S1; %no disturbence

S2=Omega2/((norm(Omega2))^2+ksi);
S22=Omega2/((norm(Omega2))+ksi);
F2=e_R2*Phi2+Psi2*P_Phi2;
A2=(R2'*R1*Omega1)'*e_R21c+(R2'*R3*Omega3)'*e_R23c;
% u20=-K(1)*Psic2*S2-K(2)*Psit2*S2-K(3)*(e_omega_2)'*e_omega_2*S2+2*K(3)*e_omega_c_2'*e_omega_t_2*S2...
%     -K(4)*F2+K(4)*Psi2*P_DF2*S2+K(4)*Phi2*A2*S2; %no disturbence
u20_nod=-K(1)*Psi2*S2-K(2)*norm(e_omega_2)*S22-K(3)*(e_omega_2)...
    -K(4)*F2+K(4)*Psi2*P_DF2*S2+K(4)*Phi2*A2*S2; %no disturbence

S3=Omega3/((norm(Omega3))^2+ksi);
S33=Omega3/((norm(Omega3))+ksi);
F3=e_R3*Phi3+Psi3*P_Phi3;
A3=(R3'*R1*Omega1)'*e_R31c+(R3'*R2*Omega2)'*e_R32c;
% u30=-K(1)*Psic3*S3-K(2)*Psit3*S3-K(3)*(e_omega_3)'*e_omega_3*S3+2*K(3)*e_omega_c_3'*e_omega_t_3*S3...
%     -K(4)*F3+K(4)*Psi3*P_DF3*S3+K(4)*Phi3*A3*S3; %no disturbence
u30_nod=-K(1)*Psi3*S3-K(2)*norm(e_omega_3)*S33-K(3)*(e_omega_3)...
    -K(4)*F3+K(4)*Psi3*P_DF3*S3+K(4)*Phi3*A3*S3; %no disturbence
end
